simulink model "bcm"  (R2020b)
settings: Solver=FixedStepDiscrete  StartTime=0.0  StopTime=10.0  FixedStep=0.1  RelTol=1e-3
libraries: simulink x1
settings Model: Creator=user32  LastModifiedBy=andvl
settings DataIOCC: ReturnWorkspaceOutputs=off
settings OptimizationCC: DefaultParameterBehavior=Inlined  PassReuseOutputArgsAs=Individual arguments  EfficientTunableParamExpr=on
settings DebuggingCC: ParameterTunabilityLossMsg=error  ArithmeticOperatorsInVariantConditions=warning
settings HardwareCC: ProdBitPerInt=16  ProdBitPerPointer=16  ProdBitPerSizeT=16  ProdBitPerPtrDiffT=16  ProdLargestAtomicFloat=None  ProdWordSize=16  ProdHWDeviceType=Atmel->AVR (8-bit)
settings SFSimCC: SimUseLocalCustomCode=off  MATLABDynamicMemAlloc=off  CustomCodeUndefinedFunction=UseInterfaceOnly
settings RTWCC: Description=Embedded Coder  SystemTargetFile=ert.tlc  TemplateMakefile=ert_default_tmf  GenerateReport=on  RTWUseLocalCustomCode=off  IncludeHyperlinkInReport=on  LaunchReport=on  GenerateTraceInfo=on  GenerateTraceReport=on  GenerateTraceReportSl=on  GenerateTraceReportSf=on  GenerateTraceReportEml=on
settings CodeAppCC: ForceParamTrailComments=on  IgnoreCustomStorageClasses=off  OperatorAnnotations=on  SimulinkDataObjDesc=on  SFDataObjDesc=on  InsertBlockDesc=on
settings ERTTargetCC: TargetLangStandard=C99 (ISO)  GenerateSampleERTMain=on  InlinedParameterPlacement=NonHierarchical  RootIOFormat=Structure reference  ERTCustomFileTemplate=example_file_process.tlc  ERTFilePackagingFormat=Compact

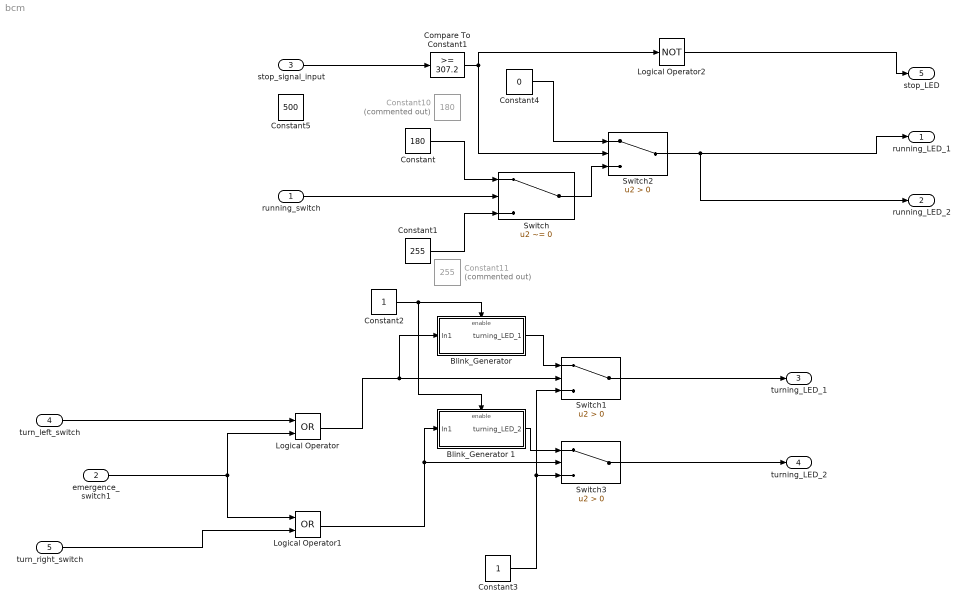
== system bcm ==
  running_switch : Inport  OutDataTypeStr=boolean
  emergence_switch1 : Inport  Port=2  OutDataTypeStr=boolean
  stop_signal_input : Inport  Port=3  OutDataTypeStr=uint16
  turn_left_switch : Inport  Port=4  OutDataTypeStr=boolean
  turn_right_switch : Inport  Port=5  OutDataTypeStr=boolean
  "Blink_Generator " : Subsystem  TreatAsAtomicUnit=on
  Blink_Generator 1 : Subsystem  TreatAsAtomicUnit=on
  Compare To Constant1 : simulink/Logic and Bit Operations/Compare To Constant  relop=>=  const=307.2  OutDataTypeStr=boolean
  Constant : Constant  Value=180  OutDataTypeStr=uint8
  Constant1 : Constant  Value=255  OutDataTypeStr=uint8
  Constant10 : Constant  Commented=on  Value=180  OutDataTypeStr=uint8
  Constant11 : Constant  Commented=on  Value=255  OutDataTypeStr=uint8
  Constant2 : Constant  OutDataTypeStr=boolean
  Constant3 : Constant  OutDataTypeStr=uint8
  Constant4 : Constant  Value=0  OutDataTypeStr=uint8
  Constant5 : Constant  Value=500
  Logical Operator : Logic  Operator=OR  AllPortsSameDT=off  OutDataTypeStr=boolean
  Logical Operator1 : Logic  Operator=OR  AllPortsSameDT=off  OutDataTypeStr=boolean
  Logical Operator2 : Logic  Operator=NOT  AllPortsSameDT=off  OutDataTypeStr=boolean
  Switch : Switch  Criteria=u2 ~= 0  Threshold=100
  Switch1 : Switch  Criteria=u2 > Threshold
  Switch2 : Switch  Criteria=u2 > Threshold
  Switch3 : Switch  Criteria=u2 > Threshold
  running_LED_1 : Outport  OutDataTypeStr=uint8  VectorParamsAs1DForOutWhenUnconnected=off
  running_LED_2 : Outport  Port=2  OutDataTypeStr=uint8  VectorParamsAs1DForOutWhenUnconnected=off
  turning_LED_1 : Outport  Port=3  OutDataTypeStr=uint8  VectorParamsAs1DForOutWhenUnconnected=off
  turning_LED_2 : Outport  Port=4  OutDataTypeStr=uint8  VectorParamsAs1DForOutWhenUnconnected=off
  stop_LED : Outport  Port=5  OutDataTypeStr=boolean
  wires:
  Switch/1 -> Switch2/3
  Constant/1 -> Switch/1
  Constant1/1 -> Switch/3
  Constant2/1 -> "Blink_Generator "/Enable, Blink_Generator 1/Enable
  Constant4/1 -> Switch2/1
  Constant3/1 -> Switch1/3, Switch3/3
  Logical Operator/1 -> "Blink_Generator "/1(In1), Switch1/2
  Logical Operator1/1 -> Blink_Generator 1/1(In1), Switch3/2
  "Blink_Generator "/1(turning_LED_1) -> Switch1/1
  Blink_Generator 1/1(turning_LED_2) -> Switch3/1
  turn_left_switch/1 -> Logical Operator/1
  emergence_switch1/1 -> Logical Operator/2, Logical Operator1/1
  turn_right_switch/1 -> Logical Operator1/2
  running_switch/1 -> Switch/2
  Switch1/1 -> turning_LED_1/1
  Switch3/1 -> turning_LED_2/1
  Switch2/1 -> running_LED_1/1, running_LED_2/1
  stop_signal_input/1 -> Compare To Constant1/1
  Compare To Constant1/1 -> Logical Operator2/1, Switch2/2
  Logical Operator2/1 -> stop_LED/1

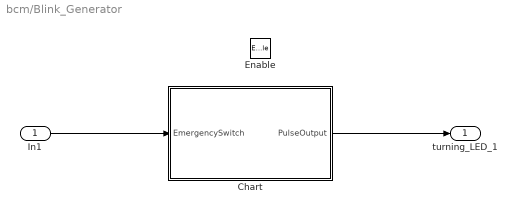
== system bcm/Blink_Generator  ==
  In1 : Inport  OutDataTypeStr=boolean
  Enable : EnablePort
  Chart : Stateflow chart  TreatAsAtomicUnit=on
  turning_LED_1 : Outport  OutDataTypeStr=uint8  VectorParamsAs1DForOutWhenUnconnected=off
  wires:
  In1/1 -> Chart/1(EmergencySwitch)
  Chart/1(PulseOutput) -> turning_LED_1/1

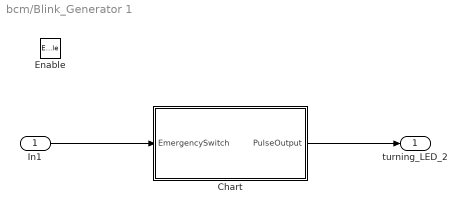
== system bcm/Blink_Generator 1 ==
  In1 : Inport  OutDataTypeStr=boolean
  Enable : EnablePort
  Chart : Stateflow chart  TreatAsAtomicUnit=on
  turning_LED_2 : Outport  OutDataTypeStr=uint8  VectorParamsAs1DForOutWhenUnconnected=off
  wires:
  In1/1 -> Chart/1(EmergencySwitch)
  Chart/1(PulseOutput) -> turning_LED_2/1

== stateflow chart bcm/Blink_Generator 1/Chart ==
  state StateHigh
    en: PulseOutput = 1;
  state StateLow
    en: PulseOutput = 0;
  (default) -> StateHigh
  StateHigh -> StateLow : [EmergencySwitch && after(50, tick)]
  StateLow -> StateHigh : [after(50, tick)]
  data: EmergencySwitch input boolean; PulseOutput output uint8

== stateflow chart bcm/Blink_Generator /Chart ==
  state StateHigh
    en: PulseOutput = 1;
  state StateLow
    en: PulseOutput = 0;
  (default) -> StateHigh
  StateHigh -> StateLow : [EmergencySwitch && after(50, tick)]
  StateLow -> StateHigh : [after(50,tick)]
  data: EmergencySwitch input boolean; PulseOutput output uint8
